simulink model "Supervisory_Logic"  (R2020b)
settings: configuration reference "freeConfigSet_Sim_ASW" (kept outside this file)
model workspace (MAT data in the model file):
  TsModel = 0.1
undefined symbols (not defined in the file): Batt_Em0_LUT, Batt_MaxCoulomb, Batt_nrCellSeries, Batt_SoC_LUT, DiscIntNeverNeededParam, SEPIC_Efficiency, voltSEPICMax
libraries: simulink x3
settings Model: ExtModeTrigDuration=8  Creator=vivekr  LastModifiedBy=vlenzi
settings ConfigSetRef: SourceName=freeConfigSet_Sim_ASW  SourceLocation=Base Workspace

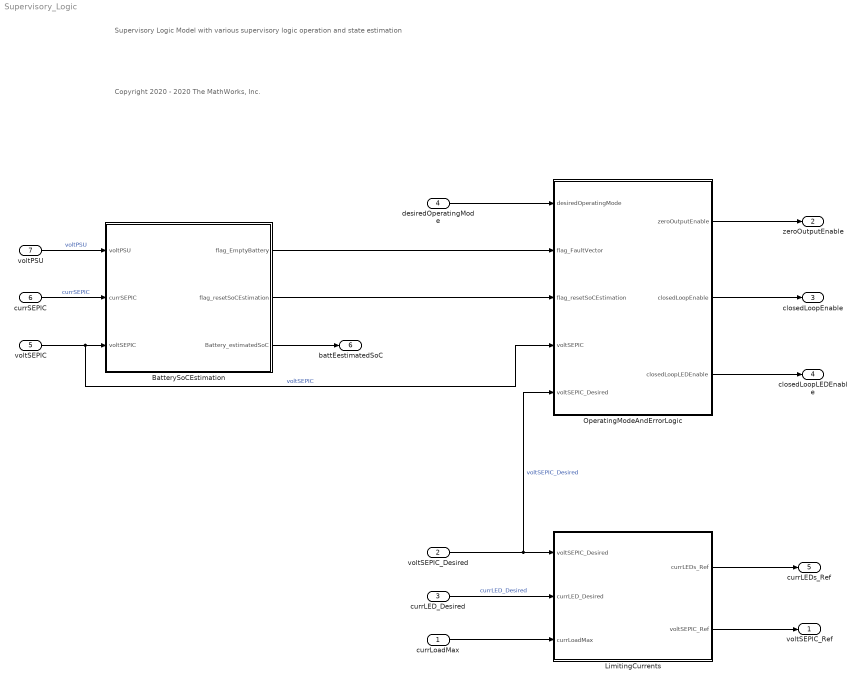
== system Supervisory_Logic ==
  note: Supervisory Logic
      | Model with various supervisory logic operation and state estimation
  note: Copyright 2020 - 2020 The MathWorks, Inc.
  currLoadMax : Inport  OutDataTypeStr=single  PortDimensions=1  SampleTime=TsModel
  voltSEPIC_Desired : Inport  Port=2  OutDataTypeStr=single  PortDimensions=1  SampleTime=TsModel
  currLED_Desired : Inport  Port=3  OutDataTypeStr=single  Unit=mA  PortDimensions=[6 1]  SampleTime=TsModel
  desiredOperatingMode : Inport  Port=4  OutDataTypeStr=Enum: operatingMode  PortDimensions=1  SampleTime=TsModel
  voltSEPIC : Inport  Port=5  OutDataTypeStr=single  Unit=V  PortDimensions=1  SampleTime=TsModel
  currSEPIC : Inport  Port=6  OutDataTypeStr=single  Unit=mA  PortDimensions=1  SampleTime=TsModel
  voltPSU : Inport  Port=7  OutDataTypeStr=single  Unit=V  PortDimensions=1  SampleTime=TsModel
  BatterySoCEstimation : Subsystem
  LimitingCurrents : Subsystem
  OperatingModeAndErrorLogic : Subsystem
  voltSEPIC_Ref : Outport  OutDataTypeStr=single  Unit=V  PortDimensions=1  SampleTime=TsModel
  zeroOutputEnable : Outport  Port=2  OutDataTypeStr=boolean  Unit=1  PortDimensions=1  SampleTime=TsModel
  closedLoopEnable : Outport  Port=3  OutDataTypeStr=boolean  Unit=1  PortDimensions=1  SampleTime=TsModel
  closedLoopLEDEnable : Outport  Port=4  OutDataTypeStr=boolean  Unit=1  PortDimensions=1  SampleTime=TsModel
  currLEDs_Ref : Outport  Port=5  OutDataTypeStr=single  Unit=mA  PortDimensions=[6 1 ]  SampleTime=TsModel
  battEestimatedSoC : Outport  Port=6  OutDataTypeStr=single  PortDimensions=1  SampleTime=TsModel
  wires:
  voltSEPIC_Desired/1 -> OperatingModeAndErrorLogic/5(voltSEPIC_Desired), LimitingCurrents/1(voltSEPIC_Desired)  "voltSEPIC_Desired"
  currLED_Desired/1 -> LimitingCurrents/2(currLED_Desired)  "currLED_Desired"
  LimitingCurrents/2(voltSEPIC_Ref) -> voltSEPIC_Ref/1
  currLoadMax/1 -> LimitingCurrents/3(currLoadMax)
  LimitingCurrents/1(currLEDs_Ref) -> currLEDs_Ref/1
  voltPSU/1 -> BatterySoCEstimation/1(voltPSU)  "voltPSU"
  currSEPIC/1 -> BatterySoCEstimation/2(currSEPIC)  "currSEPIC"
  voltSEPIC/1 -> OperatingModeAndErrorLogic/4(voltSEPIC), BatterySoCEstimation/3(voltSEPIC)  "voltSEPIC"
  BatterySoCEstimation/3(Battery_estimatedSoC) -> battEestimatedSoC/1
  desiredOperatingMode/1 -> OperatingModeAndErrorLogic/1(desiredOperatingMode)
  BatterySoCEstimation/1(flag_EmptyBattery) -> OperatingModeAndErrorLogic/2(flag_FaultVector)
  BatterySoCEstimation/2(flag_resetSoCEstimation) -> OperatingModeAndErrorLogic/3(flag_resetSoCEstimation)
  OperatingModeAndErrorLogic/1(zeroOutputEnable) -> zeroOutputEnable/1
  OperatingModeAndErrorLogic/2(closedLoopEnable) -> closedLoopEnable/1
  OperatingModeAndErrorLogic/3(closedLoopLEDEnable) -> closedLoopLEDEnable/1

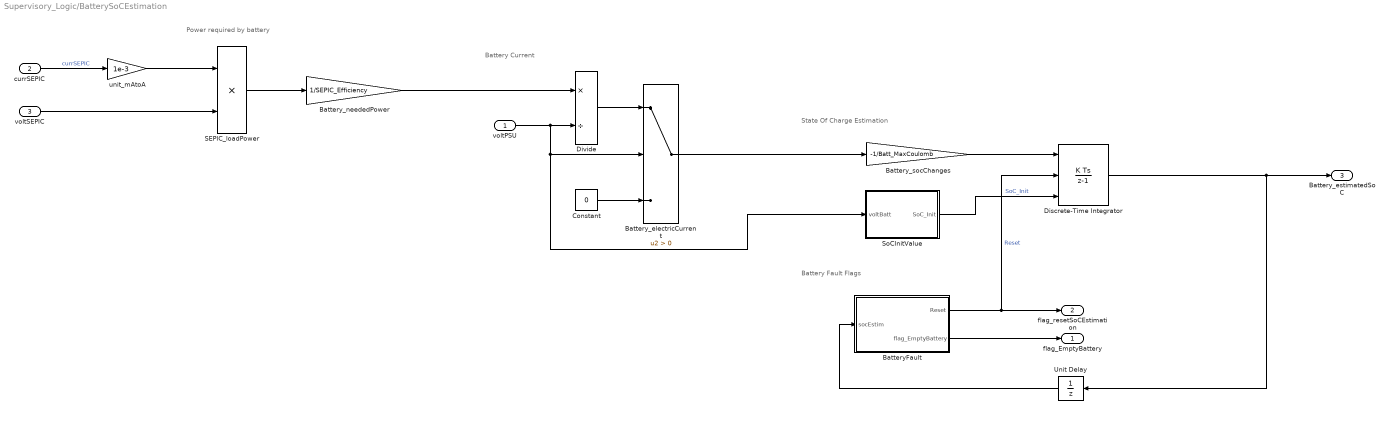
== system Supervisory_Logic/BatterySoCEstimation ==
  note: Battery Fault Flags
  note: Battery Current
  note: Power required by battery
  note: State Of Charge Estimation
  voltPSU : Inport  OutDataTypeStr=single  Unit=V  PortDimensions=1
  currSEPIC : Inport  Port=2  OutDataTypeStr=single  Unit=mA  PortDimensions=1
  voltSEPIC : Inport  Port=3
  BatteryFault : Stateflow chart  TreatAsAtomicUnit=on
  Battery_electricCurrent : Switch  Criteria=u2 > Threshold
  Battery_neededPower : Gain  Gain=1/SEPIC_Efficiency
  Battery_socChanges : Gain  Gain=-1/Batt_MaxCoulomb
  Constant : Constant  Value=0  OutDataTypeStr=single
  Discrete-Time Integrator : DiscreteIntegrator  ExternalReset=falling  InitialConditionSource=external  SampleTime=-1  OutDataTypeStr=single  LimitOutput=on  UpperSaturationLimit=1  LowerSaturationLimit=0  ICPrevOutput=DiscIntNeverNeededParam  ICPrevScaledInput=DiscIntNeverNeededParam
  Divide : Product  Inputs=*/
  SEPIC_loadPower : Product
  SoCInitValue : Subsystem  Variant=on  VariantControlMode=label  VariantControl=Variant1  LabelModeActiveChoice=Simulink_LUT
  Unit Delay : UnitDelay  SampleTime=-1  HasFrameUpgradeWarning=on
  unit_mAtoA : Gain  Gain=1e-3
  flag_EmptyBattery : Outport  OutDataTypeStr=boolean  Unit=1  PortDimensions=1  VectorParamsAs1DForOutWhenUnconnected=off
  flag_resetSoCEstimation : Outport  Port=2  OutDataTypeStr=boolean  Unit=1  PortDimensions=1  VectorParamsAs1DForOutWhenUnconnected=off
  Battery_estimatedSoC : Outport  Port=3  OutDataTypeStr=single  Unit=1  PortDimensions=1  VectorParamsAs1DForOutWhenUnconnected=off
  wires:
  Unit Delay/1 -> BatteryFault/1(socEstim)
  SoCInitValue/1(" SoC_Init") -> Discrete-Time Integrator/3  "SoC_Init"
  BatteryFault/1(Reset) -> flag_resetSoCEstimation/1, Discrete-Time Integrator/2  "Reset"
  Battery_socChanges/1 -> Discrete-Time Integrator/1
  BatteryFault/2(flag_EmptyBattery) -> flag_EmptyBattery/1
  Discrete-Time Integrator/1 -> Battery_estimatedSoC/1, Unit Delay/1
  currSEPIC/1 -> unit_mAtoA/1  "currSEPIC"
  voltSEPIC/1 -> SEPIC_loadPower/2
  SEPIC_loadPower/1 -> Battery_neededPower/1
  Battery_neededPower/1 -> Divide/1
  voltPSU/1 -> SoCInitValue/1("voltBatt "), Battery_electricCurrent/2, Divide/2
  Divide/1 -> Battery_electricCurrent/1
  Constant/1 -> Battery_electricCurrent/3
  unit_mAtoA/1 -> SEPIC_loadPower/1
  Battery_electricCurrent/1 -> Battery_socChanges/1

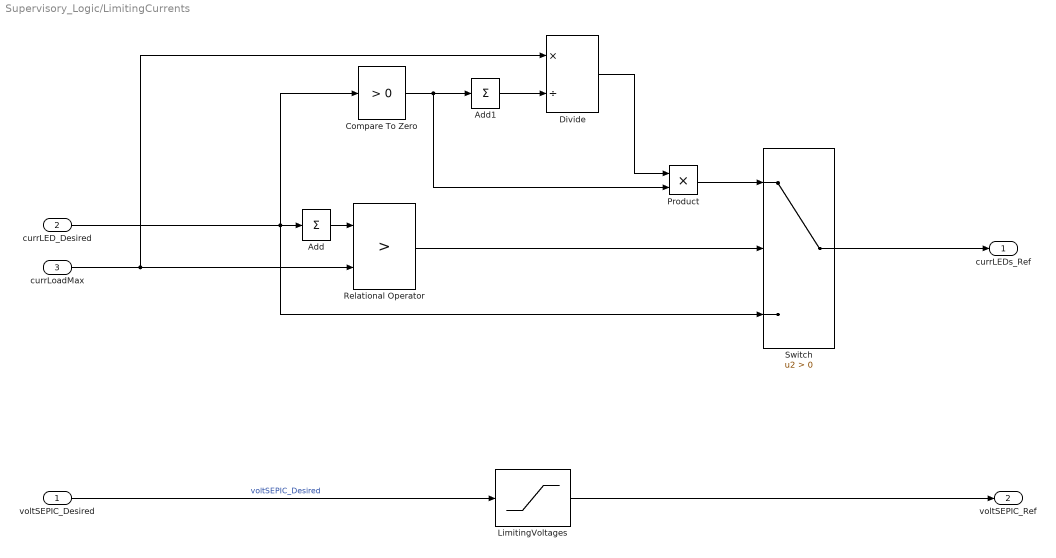
== system Supervisory_Logic/LimitingCurrents ==
  voltSEPIC_Desired : Inport  OutDataTypeStr=single  PortDimensions=1
  currLED_Desired : Inport  Port=2
  currLoadMax : Inport  Port=3
  Add : Sum  Inputs=+
  Add1 : Sum  Inputs=+
  Compare To Zero : simulink/Logic and Bit Operations/Compare To Zero  relop=>  OutDataTypeStr=boolean
  Divide : Product  Inputs=*/
  LimitingVoltages : Saturate  UpperLimit=voltSEPICMax  LowerLimit=0
  Product : Product
  Relational Operator : RelationalOperator  Operator=>  OutDataTypeStr=boolean  RndMeth=Simplest
  Switch : Switch  Criteria=u2 > Threshold
  currLEDs_Ref : Outport
  voltSEPIC_Ref : Outport  Port=2  OutDataTypeStr=single  PortDimensions=1
  wires:
  Add/1 -> Relational Operator/1
  currLED_Desired/1 -> Add/1, Compare To Zero/1, Switch/3
  currLoadMax/1 -> Relational Operator/2, Divide/1
  Relational Operator/1 -> Switch/2
  Switch/1 -> currLEDs_Ref/1
  Compare To Zero/1 -> Product/2, Add1/1
  Add1/1 -> Divide/2
  Product/1 -> Switch/1
  Divide/1 -> Product/1
  voltSEPIC_Desired/1 -> LimitingVoltages/1  "voltSEPIC_Desired"
  LimitingVoltages/1 -> voltSEPIC_Ref/1

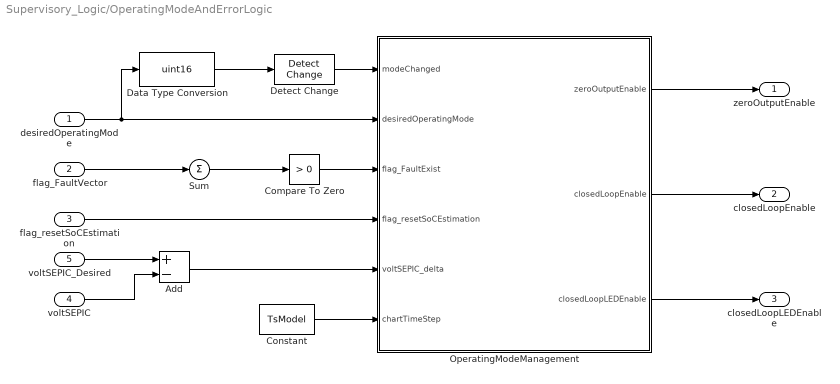
== system Supervisory_Logic/OperatingModeAndErrorLogic ==
  desiredOperatingMode : Inport
  flag_FaultVector : Inport  Port=2
  flag_resetSoCEstimation : Inport  Port=3
  voltSEPIC : Inport  Port=4
  voltSEPIC_Desired : Inport  Port=5
  Add : Sum  Inputs=+-
  Compare To Zero : simulink/Logic and Bit Operations/Compare To Zero  relop=>  OutDataTypeStr=boolean
  Constant : Constant  Value=TsModel  OutDataTypeStr=single
  Data Type Conversion : DataTypeConversion  OutDataTypeStr=uint16
  Detect Change : simulink/Logic and Bit Operations/Detect Change  vinit=0  OutDataTypeStr=boolean
  OperatingModeManagement : Stateflow chart  TreatAsAtomicUnit=on
  Sum : Sum  Inputs=+
  zeroOutputEnable : Outport  OutDataTypeStr=boolean  Unit=1  PortDimensions=1
  closedLoopEnable : Outport  Port=2  OutDataTypeStr=boolean  Unit=1  PortDimensions=1
  closedLoopLEDEnable : Outport  Port=3  OutDataTypeStr=boolean  Unit=1  PortDimensions=1
  wires:
  Compare To Zero/1 -> OperatingModeManagement/3(flag_FaultExist)
  Sum/1 -> Compare To Zero/1
  OperatingModeManagement/3(closedLoopLEDEnable) -> closedLoopLEDEnable/1
  OperatingModeManagement/2(closedLoopEnable) -> closedLoopEnable/1
  flag_resetSoCEstimation/1 -> OperatingModeManagement/4(flag_resetSoCEstimation)
  OperatingModeManagement/1(zeroOutputEnable) -> zeroOutputEnable/1
  Data Type Conversion/1 -> Detect Change/1
  Detect Change/1 -> OperatingModeManagement/1(modeChanged)
  flag_FaultVector/1 -> Sum/1
  desiredOperatingMode/1 -> Data Type Conversion/1, OperatingModeManagement/2(desiredOperatingMode)
  voltSEPIC_Desired/1 -> Add/1
  voltSEPIC/1 -> Add/2
  Add/1 -> OperatingModeManagement/5(voltSEPIC_delta)
  Constant/1 -> OperatingModeManagement/6(chartTimeStep)

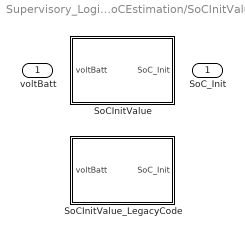
== system Supervisory_Logic/BatterySoCEstimation/SoCInitValue ==
  "voltBatt " : Inport
  SoCInitValue : Subsystem  VariantControl=Simulink_LUT
  SoCInitValue_LegacyCode : Subsystem  VariantControl=CCode_LUT
  " SoC_Init" : Outport  VectorParamsAs1DForOutWhenUnconnected=off

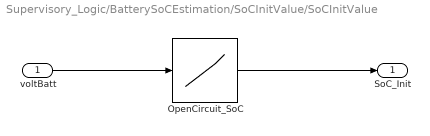
== system Supervisory_Logic/BatterySoCEstimation/SoCInitValue/SoCInitValue ==
  voltBatt : Inport
  OpenCircuit_SoC : Lookup_n-D  NumberOfTableDimensions=1  BreakpointsForDimension1=Batt_Em0_LUT*Batt_nrCellSeries  Table=Batt_SoC_LUT  InternalRulePriority=Speed  OutMin=0  OutMax=1  RndMeth=Simplest  InputSameDT=on
  SoC_Init : Outport  VectorParamsAs1DForOutWhenUnconnected=off
  wires:
  OpenCircuit_SoC/1 -> SoC_Init/1
  voltBatt/1 -> OpenCircuit_SoC/1

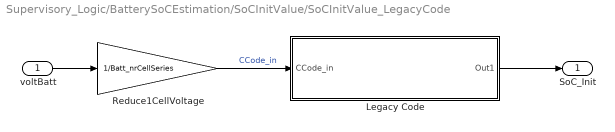
== system Supervisory_Logic/BatterySoCEstimation/SoCInitValue/SoCInitValue_LegacyCode ==
  voltBatt : Inport
  Legacy Code : Subsystem
  Reduce1CellVoltage : Gain  Gain=1/Batt_nrCellSeries
  SoC_Init : Outport  VectorParamsAs1DForOutWhenUnconnected=off
  wires:
  voltBatt/1 -> Reduce1CellVoltage/1
  Reduce1CellVoltage/1 -> Legacy Code/1(CCode_in)  "CCode_in"
  Legacy Code/1(Out1) -> SoC_Init/1

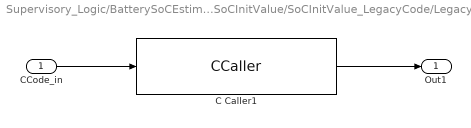
== system Supervisory_Logic/BatterySoCEstimation/SoCInitValue/SoCInitValue_LegacyCode/Legacy Code ==
  CCode_in : Inport
  C Caller1 : CCaller  FunctionName=EmLiIon_LUT  PortSpecificationStruct="%)30     .    R ,   8    (     @         %    \"     (    !     0         %  0 \"0    $    _    07)G3F%M90  4&]R=$YA;64 4V-O<&4     26YD97@     5'EP90      4VEZ90      27-';&]B86P   X    P    !@    @    $          4    (     0    ,    !         !   P!O=70 #@   #     &    \"     0         !0    @    !     P    $         $  # &]U=  .    .     8    (    !          %    \"     $    &     0         0    !@   $]U='!U=   #@   #@    &    \"     8         !0    @    !     0    $         \"0    @               X    X    !@    @    $          4    (     0    8    !         !     &    <VEN9VQE   .    ,     8    (    !          %    \"     $    !     0         0  $ ,0    X    P    !@    @    ) @        4    (     0    $    !          (  0      #@   #@    &    \"     0         !0    @    !    !0    $         $     4   !I;G!U=     X    X    !@    @    $          4    (     0    4    !         !     %    :6YP=70    .    .     8    (    !          %    \"     $    %     0         0    !0   $EN<'5T    #@   #@    &    \"     8         !0    @    !     0    $         \"0    @               X    X    !@    @    $          4    (     0    8    !         !     &    <VEN9VQE   .    ,     8    (    !          %    \"     $    !     0         0  $ ,0    X    P    !@    @    ) @        4    (     0    $    !          (  0"
  Out1 : Outport  VectorParamsAs1DForOutWhenUnconnected=off
  wires:
  C Caller1/1 -> Out1/1
  CCode_in/1 -> C Caller1/1

== stateflow chart Supervisory_Logic/BatterySoCEstimation/BatteryFault ==
  state Resetting_Integrator
    en:Reset=true;
    flag_EmptyBattery=false;
    ex:Reset=false;
  state running
    state Normal
      du:flag_EmptyBattery=false;
    state Battery_Empty
      en:flag_EmptyBattery=true;
    (default) -> Normal
    Normal -> Battery_Empty : [socEstim<=0.05]
  (default) -> Resetting_Integrator
  Resetting_Integrator -> running : [after(3,sec)]
  data: Reset output boolean; socEstim input single size=1; flag_EmptyBattery output

== stateflow chart Supervisory_Logic/OperatingModeAndErrorLogic/OperatingModeManagement ==
  state Operation
    state OperatingMode [parallel]
      settings: executionOrder=2
      state AllOpenLoop
        en:closedLoopEnable=false;
        en:closedLoopLEDEnable=false;
      state VoltOpen_CurrClosed
        en:closedLoopEnable=false;
        en:closedLoopLEDEnable=true;
      state VoltClosed_CurrOpen
        en:closedLoopEnable=true;
        en:closedLoopLEDEnable=false;
      state AllClosedLoop
        en:closedLoopEnable=true;
        en:closedLoopLEDEnable=true;
      state AutomaticOperation
        state AllOpenLoop
          en:closedLoopEnable=false;
          en:closedLoopLEDEnable=false;
          en:counter=0;
        state WaitingForVoltageSettling
          en:closedLoopEnable=false;
          en:closedLoopLEDEnable=false;
          du:counter=counter+1;
        state AllClosedLoop
          en:closedLoopEnable=true;
          en:closedLoopLEDEnable=true;
        (default) -> Operation.OperatingMode.AutomaticOperation.AllOpenLoop
        Operation.OperatingMode.AutomaticOperation.AllOpenLoop -> WaitingForVoltageSettling : [abs(voltSEPIC_delta) <=1]
        WaitingForVoltageSettling -> Operation.OperatingMode.AutomaticOperation.AllOpenLoop [order 2] : [abs(voltSEPIC_delta) >1.5]
        WaitingForVoltageSettling -> Operation.OperatingMode.AutomaticOperation.AllClosedLoop [order 1] : [counter>floor(2/chartTimeStep)]
      state NoOutput
        en:zeroOutputEnable=true;
      (default) -> (junction 91)
      (junction 91) -> Operation.OperatingMode.AllOpenLoop [order 1] : [desiredOperatingMode==AllOpenLoop]
      Operation.OperatingMode.AllOpenLoop -> OperatingMode : [modeChanged]
      (junction 91) -> (junction 92) [order 2]
      (junction 92) -> VoltOpen_CurrClosed [order 1] : [desiredOperatingMode==VoltOpen_CurrClosed]
      VoltOpen_CurrClosed -> OperatingMode : [modeChanged]
      (junction 92) -> (junction 93) [order 2]
      VoltClosed_CurrOpen -> OperatingMode : [modeChanged]
      (junction 93) -> VoltClosed_CurrOpen [order 1] : [desiredOperatingMode==VoltClosed_CurrOpen]
      (junction 93) -> (junction 94) [order 2]
      (junction 94) -> Operation.OperatingMode.AllClosedLoop [order 1] : [desiredOperatingMode==AllClosedLoop]
      Operation.OperatingMode.AllClosedLoop -> OperatingMode : [modeChanged]
      (junction 94) -> (junction 127) [order 2]
      (junction 127) -> AutomaticOperation [order 1] : [desiredOperatingMode==AutomaticOperation]
      (junction 127) -> NoOutput [order 2]
      AutomaticOperation -> OperatingMode : [modeChanged]
      NoOutput -> OperatingMode : [modeChanged]
    state CheckingFault [parallel]
      settings: executionOrder=1
      state SystemKO
        en:zeroOutputEnable=true;
      state SystemOK
        en:zeroOutputEnable=false;
      (default) -> SystemKO
      SystemOK -> SystemKO : [flag_FaultExist]
      SystemKO -> SystemOK : [~flag_FaultExist]
  state Initialization_no_output
    en:closedLoopEnable=false;
    en:closedLoopLEDEnable=false;
    en:zeroOutputEnable=true;
  (default) -> Initialization_no_output
  Initialization_no_output -> Operation : [desiredOperatingMode ~= NoOutput &&flag_resetSoCEstimation==0 ]
  data: modeChanged input boolean; zeroOutputEnable output boolean size=1; desiredOperatingMode input Enum: operatingMode; closedLoopEnable output boolean size=1; closedLoopLEDEnable output boolean size=1; flag_FaultExist input boolean; flag_resetSoCEstimation input boolean; voltSEPIC_delta input; chartTimeStep input; counter local
